simulink model "Ultrasonic_Control_slave"  (R2017b)
settings: Solver=FixedStepDiscrete  StartTime=0.0  StopTime=10  FixedStep=dt  RelTol=1e-3
InitFcn:
  | mbd_s32k14_consistency_checks(bdroot(gcs));
model workspace (MAT data in the model file):
  dt = Simulink.Parameter
  dt.Value = 0.01
  dt.DataType = 'auto'
  dt.Dimensions = [1 1]
undefined symbols (not defined in the file): B8, C7, D1, D2, G3, PTC6, PTC7, PTD15, PTE4, PTE5
libraries: mbd_s32k14_ec_toolbox x19
Description:
  | BLDC FOC Control example for S32K144EVB-Q100 and MotorGD
  | This model is designed and tuned to work with Linix BLDC motor (hall sensors and 2 pole pairs)
  | 
  | Features:
  | - Motor Speed Reference read via SW3 (increment) and SW2 (decrement)
  | - Motor can rotate CW (default) or CCW based on SW3/2 values
  | - Read DC voltage/current based on PWM trigger signal and PDB-ADC HW interrupts
  | 
  | HW and SW setup:
  | - Configure S32K144EVB-Q100: place R168 and remove R167 (HALL A signal routing), and place R166 and remove R165 (HALL B signal routing)
  | - Plug in DEVKIT MOTORGD into S32K144EVB
  | - Connect the motor phases to MOTORGD J13 connector (i.e. Linix Motor - phA-white/phB-blue/phC-green)
  | - Connect the Hall Sensors on JP1 connector
  | - Power on the MOTORGD via J7 connector
  | 
  | Validation:
  | - Motor should start rotating at 1000 rpm.
  | - Use FreeMASTER project to vizualize different parameters
  | 
  | Copyright (c) 2017 NXP
  | version 3.0.0
settings Model: Creator=B21307  LastModifiedBy=sarad
settings DataIOCC: ExternalInput=off  InitialState=off  SaveOutput=off  SignalLogging=off  SaveTime=off
settings OptimizationCC: DefaultParameterBehavior=Inlined  UseFloatMulNetSlope=on  UseSpecifiedMinMax=on  InlineInvariantSignals=on  ZeroExternalMemoryAtStartup=off  ZeroInternalMemoryAtStartup=off  NoFixptDivByZeroProtection=on  EfficientFloat2IntCast=on  LifeSpan=1  SimCompilerOptimization=on
settings DebuggingCC: ArrayBoundsChecking=error  SignalInfNanChecking=error  WriteAfterWriteMsg=EnableAllAsError  WriteAfterReadMsg=EnableAllAsError  SaveWithDisabledLinksMsg=error  InheritedTsInSrcMsg=none  SingleTaskRateTransMsg=error  TasksWithSamePriorityMsg=error  SigSpecEnsureSampleTimeMsg=error  ParameterPrecisionLossMsg=none  ParameterTunabilityLossMsg=error  VectorMatrixConversionMsg=warning  SignalLabelMismatchMsg=warning  UnconnectedInputMsg=error  UnconnectedOutputMsg=error  UnconnectedLineMsg=error  UniqueDataStoreMsg=error  AssertControl=EnableAll  AllowSymbolicDim=off  ModelReferenceIOMsg=warning  ModelReferenceVersionMismatchMessage=warning  ModelReferenceIOMismatchMessage=warning  UnknownTsInhSupMsg=error  SFUnusedDataAndEventsDiag=error  SFInvalidInputDataAccessInChartInitDiag=error  SFTransitionOutsideNaturalParentDiag=error  SFUnreachableExecutionPathDiag=error  SFUndirectedBroadcastEventsDiag=error  SFTransitionActionBeforeConditionDiag=error  SFExecutionAtInitializationDiag=none
settings HardwareCC: ProdBitPerPointer=32  ProdBitPerSizeT=32  ProdBitPerPtrDiffT=32  ProdLargestAtomicInteger=Long  ProdLargestAtomicFloat=Double  ProdWordSize=32  ProdHWDeviceType=ARM Compatible->ARM Cortex
settings ModelReferenceCC: UpdateModelReferenceTargets=Force
settings SFSimCC: MATLABDynamicMemAlloc=off
settings RTWCC: SystemTargetFile=mbd_s32k14.tlc  MakeCommand=mbd_s32k14_make_rtw COPY_MDLREF_INCLUDES=0  TemplateMakefile=mbd_s32k14.tmf  Description=Model Based Design Toolbox S32K14x Code Generation Target
settings CodeAppCC: ForceParamTrailComments=on  IgnoreCustomStorageClasses=off  OperatorAnnotations=on  SimulinkDataObjDesc=on  SFDataObjDesc=on  MATLABFcnDesc=on  InsertBlockDesc=on  StateflowObjectComments=on  MATLABSourceComments=on  ReqsInCode=on
settings STFCustomTargetCC: CombineOutputUpdateFcns=on  ERTCustomFileBanners=on  SupportContinuousTime=off  SupportNonInlinedSFcns=off  RemoveResetFunc=on  MATLABClassNameForMDSCustomization=Simulink.SoftwareTarget.ERTCustomization  GRTInterface=off  SystemTargetFile=mbd_s32k14.tlc
settings ERTTargetCC: MultiwordLength=2048  ParMdlRefBuildCompliant=off  CompOptLevelCompliant=off  ConcurrentExecutionCompliant=off  ModelStepFunctionPrototypeControlCompliant=off  CPPClassGenCompliant=off  UseToolchainInfoCompliant=off  InlinedParameterPlacement=NonHierarchical  ERTCustomFileTemplate=example_file_process.tlc  ConvertIfToSwitch=off  SuppressUnreachableDefaultCases=off

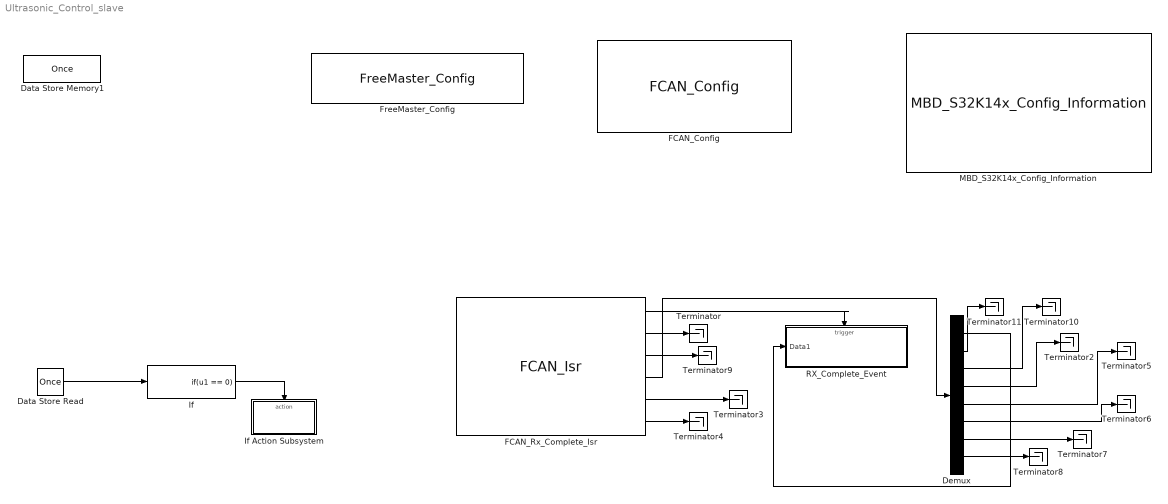
== system Ultrasonic_Control_slave ==
  Data Store Memory1 : DataStoreMemory  DataStoreName=Once  ReadBeforeWriteMsg=warning  WriteAfterWriteMsg=warning  WriteAfterReadMsg=warning  ShowAdditionalParam=off  OutDataTypeStr=uint32
  Data Store Read : DataStoreRead  DataStoreName=Once
  Demux : Demux  Outputs=8
  FCAN_Config : mbd_s32k14_ec_toolbox/S32K14x/Communication Blocks/Flex CAN Blocks/FCAN_Config  Priority=1  can_instance=0  can_mode=Normal mode  can_max_num_mb=16  can_rx=PTE4 : [9] : [6] : [D1]  can_tx=PTE5 : [8] : [5] : [D2]  show_adv_opts=on  can_clk_src=Peripheral clock  can_presdiv=9  can_rjw=0  can_pseg1=3  can_pseg2=3  can_propseg=6  can_cbt_presdiv=9  can_cbt_rjw=0  can_cbt_pseg1=3  can_cbt_pseg2=3  can_cbt_propseg=6  can_fd_enable=on  can_payload=8  can_rxfifo_enable=off  can_fifo_id_filter_extended=off  can_fifo_id_filter_remote=off  can_num_id_filters=8  can_fifo_id_format=A  can_fifo_id_filter={'0x0', '0x0', '0x0', '0x0', '0x0', '0x0', '0x0', '0x0'}  can_pn_enable=off  can_wakeup_match=off  can_wakeup_timeout=off  can_timeout_en=off  can_match_timeout=1  can_multiple_matches_en=off  can_num_matches=1  can_idfilter_extendedid=off  can_idfilter_remoteframe=off  can_idfilter_type=Match exact  can_idfilter_id1=0  can_idfilter_id2=0  can_payloadfilter_enable=off  can_payloadfilter_dlclow=0  can_payloadfilter_dlchigh=0  can_payloadfilter_type=Match exact  can_payloadfilter_payload1_b0=0  can_payloadfilter_payload1_b1=0  can_payloadfilter_payload1_b2=0  can_payloadfilter_payload1_b3=0  can_payloadfilter_payload1_b4=0  can_payloadfilter_payload1_b5=0  can_payloadfilter_payload1_b6=0  can_payloadfilter_payload1_b7=0  can_payloadfilter_payload2_b0=0  can_payloadfilter_payload2_b1=0  can_payloadfilter_payload2_b2=0  can_payloadfilter_payload2_b3=0  can_payloadfilter_payload2_b4=0  can_payloadfilter_payload2_b5=0  can_payloadfilter_payload2_b6=0  can_payloadfilter_payload2_b7=0
  FCAN_Rx_Complete_Isr : mbd_s32k14_ec_toolbox/S32K14x/Communication Blocks/Flex CAN Blocks/FCAN_Isr  can_instance=0  can_event=Rx Complete
  FreeMaster_Config : mbd_s32k14_ec_toolbox/S32K14x/Utility Blocks/FreeMaster_Config  interface=UART1  baudrate=115200  rxd=PTC6 : [81] : [52] : [C7]  txd=PTC7 : [80] : [51] : [B8]  mode=Short Interrupt  isr_prio=3  show_adv_opts=on  use_scope=on  max_scope_vars=8  use_recorder=on  max_rec_vars=8  rec_buff_size=1024  rec_timebase=0 milliseconds  comm_buffer_size_auto=on  comm_buffer_size=255  comm_rqueue_size_default=on  comm_rqueue_size=32
  If : If  IfExpression=u1 == 0  ShowElse=off
  If Action Subsystem : Subsystem  TreatAsAtomicUnit=on
  MBD_S32K14x_Config_Information : mbd_s32k14_ec_toolbox/S32K14x/MBD_S32K14x_Config_Information  disp_str=|  config_params=[]
      | Target : S32K144-64KB_SRAM
      | Package : 100-pin
      | System clock : 80 MHz
      | XTAL clock : External 8 MHz
      | Compiler : GCC
      | Target Type : FLASH
      | Download Code after build : (OpenSDA: E)
      | Step Tick Interrupt Priority : 15
  RX_Complete_Event : Subsystem  TreatAsAtomicUnit=on
      settings: RTWSystemCode=Nonreusable function
  Terminator{,2..11} (11 alike) : Terminator
  wires:
  Demux/8 -> Terminator8/1
  Demux/1 -> RX_Complete_Event/1(Data1)
  FCAN_Rx_Complete_Isr/3 -> Terminator9/1
  Demux/6 -> Terminator6/1
  FCAN_Rx_Complete_Isr/2 -> Terminator/1
  Demux/7 -> Terminator7/1
  Demux/5 -> Terminator5/1
  FCAN_Rx_Complete_Isr/1 -> RX_Complete_Event/Trigger
  FCAN_Rx_Complete_Isr/4 -> Demux/1
  FCAN_Rx_Complete_Isr/5 -> Terminator3/1
  FCAN_Rx_Complete_Isr/6 -> Terminator4/1
  Demux/2 -> Terminator11/1
  Demux/3 -> Terminator10/1
  Demux/4 -> Terminator2/1
  Data Store Read/1 -> If/1
  If/1 -> If Action Subsystem/Action

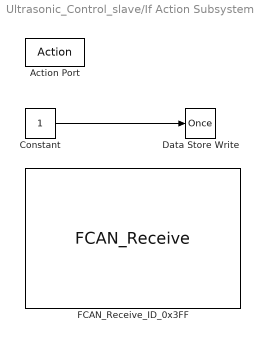
== system Ultrasonic_Control_slave/If Action Subsystem ==
  Action Port : ActionPort  ActionType=then
  Constant : Constant  OutDataTypeStr=uint32
  Data Store Write : DataStoreWrite  DataStoreName=Once
  FCAN_Receive_ID_0x3FF : mbd_s32k14_ec_toolbox/S32K14x/Communication Blocks/Flex CAN Blocks/FCAN_Receive  can_instance=0  can_mode=Non-blocking  can_timeout_ms=0  can_mb_idx=14  can_extended_id=off  can_is_remote=off  can_id=3FF  can_msg_mask=FFFFFFFF  show_adv_opts=on  can_use_rxfifo=off  can_fd_enable=on
  wires:
  Constant/1 -> Data Store Write/1

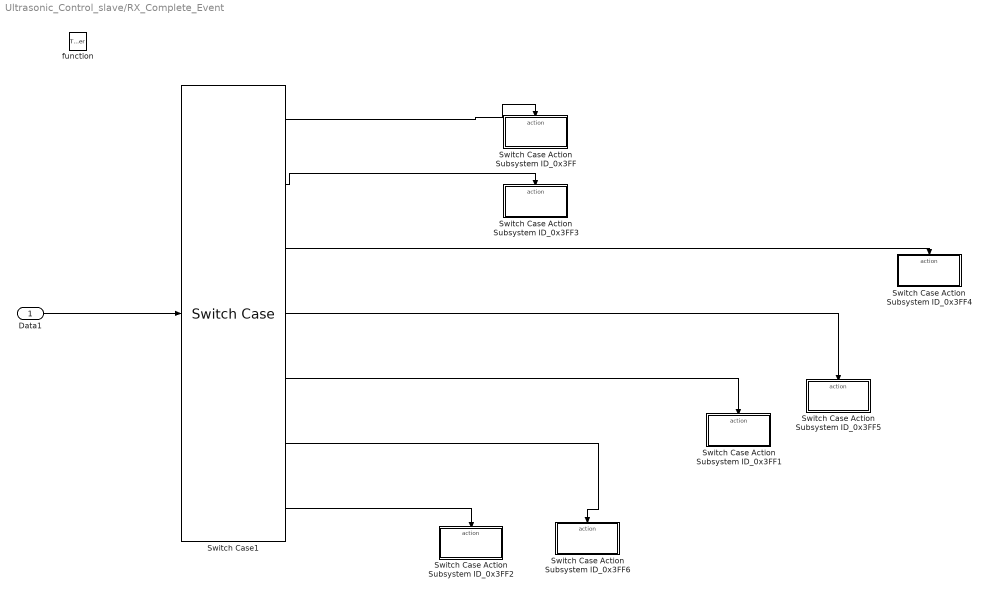
== system Ultrasonic_Control_slave/RX_Complete_Event ==
  Data1 : Inport
  function : TriggerPort  TriggerType=function-call  VariantControl=(inherit)
  Switch Case Action Subsystem ID_0x3FF : Subsystem  TreatAsAtomicUnit=on
  Switch Case Action Subsystem ID_0x3FF1 : Subsystem  TreatAsAtomicUnit=on
  Switch Case Action Subsystem ID_0x3FF2 : Subsystem  TreatAsAtomicUnit=on
  Switch Case Action Subsystem ID_0x3FF3 : Subsystem  TreatAsAtomicUnit=on
  Switch Case Action Subsystem ID_0x3FF4 : Subsystem  TreatAsAtomicUnit=on
  Switch Case Action Subsystem ID_0x3FF5 : Subsystem  TreatAsAtomicUnit=on
  Switch Case Action Subsystem ID_0x3FF6 : Subsystem  TreatAsAtomicUnit=on
  Switch Case1 : SwitchCase  CaseConditions={hex2dec('030'),hex2dec('031'),hex2dec('032'),hex2dec('033'),hex2dec('034'),hex2dec('035'),hex2dec('036')}  ShowDefaultCase=off
  wires:
  Switch Case1/2 -> Switch Case Action Subsystem ID_0x3FF3/Action
  Switch Case1/5 -> Switch Case Action Subsystem ID_0x3FF1/Action
  Switch Case1/6 -> Switch Case Action Subsystem ID_0x3FF6/Action
  Switch Case1/4 -> Switch Case Action Subsystem ID_0x3FF5/Action
  Switch Case1/1 -> Switch Case Action Subsystem ID_0x3FF/Action
  Switch Case1/3 -> Switch Case Action Subsystem ID_0x3FF4/Action
  Data1/1 -> Switch Case1/1
  Switch Case1/7 -> Switch Case Action Subsystem ID_0x3FF2/Action

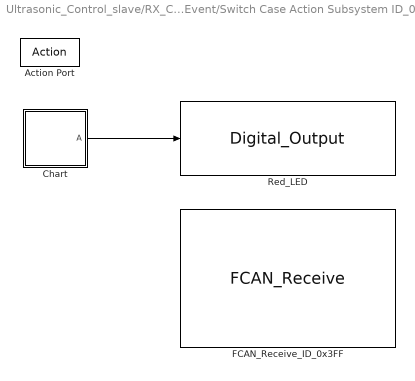
== system Ultrasonic_Control_slave/RX_Complete_Event/Switch Case Action Subsystem ID_0x3FF ==
  Action Port : ActionPort  ActionType=case
  Chart : Stateflow chart  TreatAsAtomicUnit=on
  FCAN_Receive_ID_0x3FF : mbd_s32k14_ec_toolbox/S32K14x/Communication Blocks/Flex CAN Blocks/FCAN_Receive  can_instance=0  can_mode=Non-blocking  can_timeout_ms=0  can_mb_idx=14  can_extended_id=off  can_is_remote=off  can_id=3FF  can_msg_mask=FFFFFFFF  show_adv_opts=on  can_use_rxfifo=off  can_fd_enable=on
  Red_LED : mbd_s32k14_ec_toolbox/S32K14x/Peripheral Interface Blocks/Digital_Output  gpio_pin=PTD15 : [22] : [15] : [G3]  port=D  pin=15  drive_strength=Low  slew_rate=Fast
  wires:
  Chart/1(" A") -> Red_LED/1

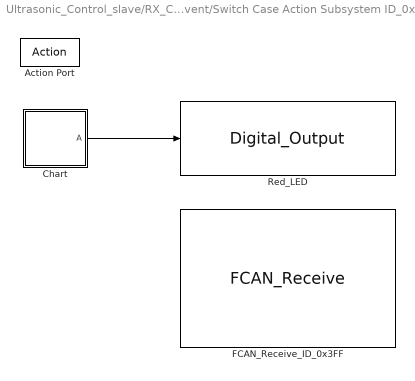
== system Ultrasonic_Control_slave/RX_Complete_Event/Switch Case Action Subsystem ID_0x3FF1 ==
  Action Port : ActionPort  ActionType=case
  Chart : Stateflow chart  TreatAsAtomicUnit=on
  FCAN_Receive_ID_0x3FF : mbd_s32k14_ec_toolbox/S32K14x/Communication Blocks/Flex CAN Blocks/FCAN_Receive  can_instance=0  can_mode=Non-blocking  can_timeout_ms=0  can_mb_idx=14  can_extended_id=off  can_is_remote=off  can_id=3FF  can_msg_mask=FFFFFFFF  show_adv_opts=on  can_use_rxfifo=off  can_fd_enable=on
  Red_LED : mbd_s32k14_ec_toolbox/S32K14x/Peripheral Interface Blocks/Digital_Output  gpio_pin=PTD15 : [22] : [15] : [G3]  port=D  pin=15  drive_strength=Low  slew_rate=Fast
  wires:
  Chart/1(" A") -> Red_LED/1

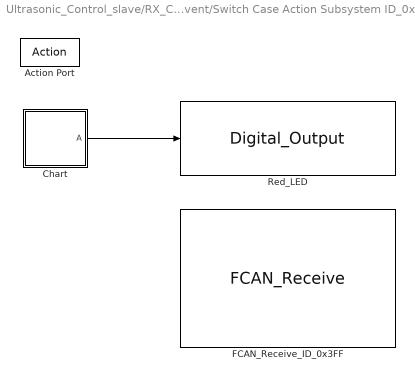
== system Ultrasonic_Control_slave/RX_Complete_Event/Switch Case Action Subsystem ID_0x3FF2 ==
  Action Port : ActionPort  ActionType=case
  Chart : Stateflow chart  TreatAsAtomicUnit=on
  FCAN_Receive_ID_0x3FF : mbd_s32k14_ec_toolbox/S32K14x/Communication Blocks/Flex CAN Blocks/FCAN_Receive  can_instance=0  can_mode=Non-blocking  can_timeout_ms=0  can_mb_idx=14  can_extended_id=off  can_is_remote=off  can_id=3FF  can_msg_mask=FFFFFFFF  show_adv_opts=on  can_use_rxfifo=off  can_fd_enable=on
  Red_LED : mbd_s32k14_ec_toolbox/S32K14x/Peripheral Interface Blocks/Digital_Output  gpio_pin=PTD15 : [22] : [15] : [G3]  port=D  pin=15  drive_strength=Low  slew_rate=Fast
  wires:
  Chart/1(" A") -> Red_LED/1

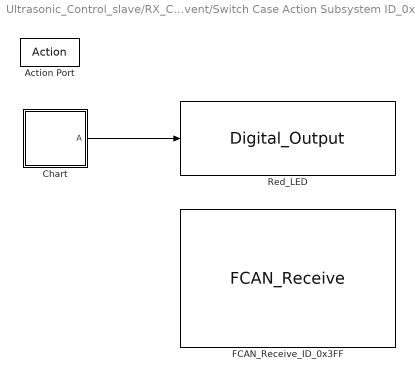
== system Ultrasonic_Control_slave/RX_Complete_Event/Switch Case Action Subsystem ID_0x3FF3 ==
  Action Port : ActionPort  ActionType=case
  Chart : Stateflow chart  TreatAsAtomicUnit=on
  FCAN_Receive_ID_0x3FF : mbd_s32k14_ec_toolbox/S32K14x/Communication Blocks/Flex CAN Blocks/FCAN_Receive  can_instance=0  can_mode=Non-blocking  can_timeout_ms=0  can_mb_idx=14  can_extended_id=off  can_is_remote=off  can_id=3FF  can_msg_mask=FFFFFFFF  show_adv_opts=on  can_use_rxfifo=off  can_fd_enable=on
  Red_LED : mbd_s32k14_ec_toolbox/S32K14x/Peripheral Interface Blocks/Digital_Output  gpio_pin=PTD15 : [22] : [15] : [G3]  port=D  pin=15  drive_strength=Low  slew_rate=Fast
  wires:
  Chart/1(" A") -> Red_LED/1

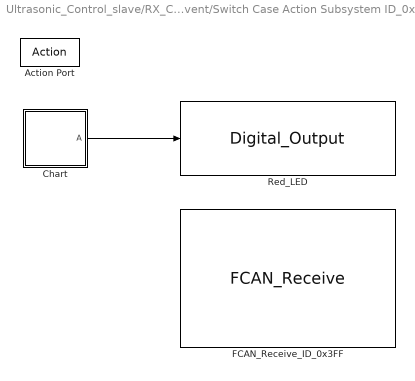
== system Ultrasonic_Control_slave/RX_Complete_Event/Switch Case Action Subsystem ID_0x3FF4 ==
  Action Port : ActionPort  ActionType=case
  Chart : Stateflow chart  TreatAsAtomicUnit=on
  FCAN_Receive_ID_0x3FF : mbd_s32k14_ec_toolbox/S32K14x/Communication Blocks/Flex CAN Blocks/FCAN_Receive  can_instance=0  can_mode=Non-blocking  can_timeout_ms=0  can_mb_idx=14  can_extended_id=off  can_is_remote=off  can_id=3FF  can_msg_mask=FFFFFFFF  show_adv_opts=on  can_use_rxfifo=off  can_fd_enable=on
  Red_LED : mbd_s32k14_ec_toolbox/S32K14x/Peripheral Interface Blocks/Digital_Output  gpio_pin=PTD15 : [22] : [15] : [G3]  port=D  pin=15  drive_strength=Low  slew_rate=Fast
  wires:
  Chart/1(" A") -> Red_LED/1

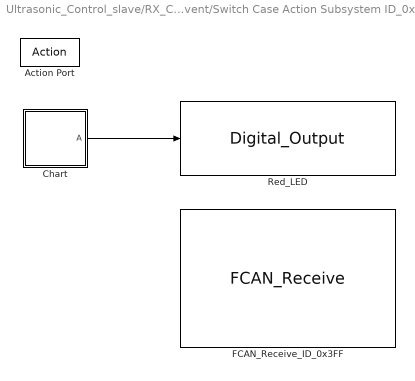
== system Ultrasonic_Control_slave/RX_Complete_Event/Switch Case Action Subsystem ID_0x3FF5 ==
  Action Port : ActionPort  ActionType=case
  Chart : Stateflow chart  TreatAsAtomicUnit=on
  FCAN_Receive_ID_0x3FF : mbd_s32k14_ec_toolbox/S32K14x/Communication Blocks/Flex CAN Blocks/FCAN_Receive  can_instance=0  can_mode=Non-blocking  can_timeout_ms=0  can_mb_idx=14  can_extended_id=off  can_is_remote=off  can_id=3FF  can_msg_mask=FFFFFFFF  show_adv_opts=on  can_use_rxfifo=off  can_fd_enable=on
  Red_LED : mbd_s32k14_ec_toolbox/S32K14x/Peripheral Interface Blocks/Digital_Output  gpio_pin=PTD15 : [22] : [15] : [G3]  port=D  pin=15  drive_strength=Low  slew_rate=Fast
  wires:
  Chart/1(" A") -> Red_LED/1

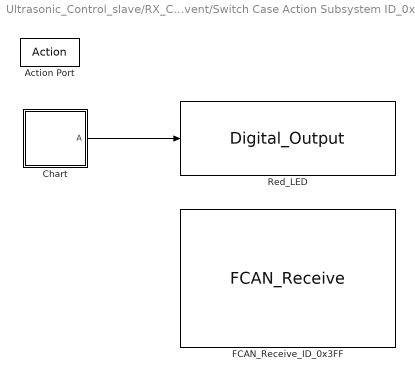
== system Ultrasonic_Control_slave/RX_Complete_Event/Switch Case Action Subsystem ID_0x3FF6 ==
  Action Port : ActionPort  ActionType=case
  Chart : Stateflow chart  TreatAsAtomicUnit=on
  FCAN_Receive_ID_0x3FF : mbd_s32k14_ec_toolbox/S32K14x/Communication Blocks/Flex CAN Blocks/FCAN_Receive  can_instance=0  can_mode=Non-blocking  can_timeout_ms=0  can_mb_idx=14  can_extended_id=off  can_is_remote=off  can_id=3FF  can_msg_mask=FFFFFFFF  show_adv_opts=on  can_use_rxfifo=off  can_fd_enable=on
  Red_LED : mbd_s32k14_ec_toolbox/S32K14x/Peripheral Interface Blocks/Digital_Output  gpio_pin=PTD15 : [22] : [15] : [G3]  port=D  pin=15  drive_strength=Low  slew_rate=Fast
  wires:
  Chart/1(" A") -> Red_LED/1

== stateflow chart Ultrasonic_Control_slave/RX_Complete_Event/Switch Case Action Subsystem ID_0x3FF/Chart ==
  state A
  state A1
  (default) -> A
  A -> A1
  A1 -> A
  data: A output boolean [0..1]

== stateflow chart Ultrasonic_Control_slave/RX_Complete_Event/Switch Case Action Subsystem ID_0x3FF4/Chart ==
  state A
  state A1
  (default) -> A
  A -> A1
  A1 -> A
  data: A output boolean [0..1]

== stateflow chart Ultrasonic_Control_slave/RX_Complete_Event/Switch Case Action Subsystem ID_0x3FF1/Chart ==
  state A
  state A1
  (default) -> A
  A -> A1
  A1 -> A
  data: A output boolean [0..1]

== stateflow chart Ultrasonic_Control_slave/RX_Complete_Event/Switch Case Action Subsystem ID_0x3FF2/Chart ==
  state A
  state A1
  (default) -> A
  A -> A1
  A1 -> A
  data: A output boolean [0..1]

== stateflow chart Ultrasonic_Control_slave/RX_Complete_Event/Switch Case Action Subsystem ID_0x3FF3/Chart ==
  state A
  state A1
  (default) -> A
  A -> A1
  A1 -> A
  data: A output boolean [0..1]

== stateflow chart Ultrasonic_Control_slave/RX_Complete_Event/Switch Case Action Subsystem ID_0x3FF5/Chart ==
  state A
  state A1
  (default) -> A
  A -> A1
  A1 -> A
  data: A output boolean [0..1]

== stateflow chart Ultrasonic_Control_slave/RX_Complete_Event/Switch Case Action Subsystem ID_0x3FF6/Chart ==
  state A
  state A1
  (default) -> A
  A -> A1
  A1 -> A
  data: A output boolean [0..1]
